simulink model "ModellierungMotor"  (R2014a)
settings: Solver=ode45  StartTime=0.0  StopTime=50  RelTol=1e-3
values from neighbouring files (symbols this model uses):
  Idea = [100000;100]    [DelayDensity_GeneticAlgorithm.m]
  System_A = [0 1 0;0 0 1;0 -C/A -B/A]    [DelayDensity_GeneticAlgorithm.m]
  System_B = [0;0;1/A]    [DelayDensity_GeneticAlgorithm.m]
  System_C = [1 0 0]    [DelayDensity_GeneticAlgorithm.m]
  System_S1 = [0;0;S1/A]    [DelayDensity_GeneticAlgorithm.m]
  System_S2 = [0;0;S2/A]    [DelayDensity_GeneticAlgorithm.m]
  V = -1/(System_C*inv(System_A-System_B*K)*System_B)    [DelayDensity_GeneticAlgorithm.m]
undefined symbols (not defined in the file or in its folder): K, PD, PI, PK
settings Model: Creator=shenc  LastModifiedBy=shenc

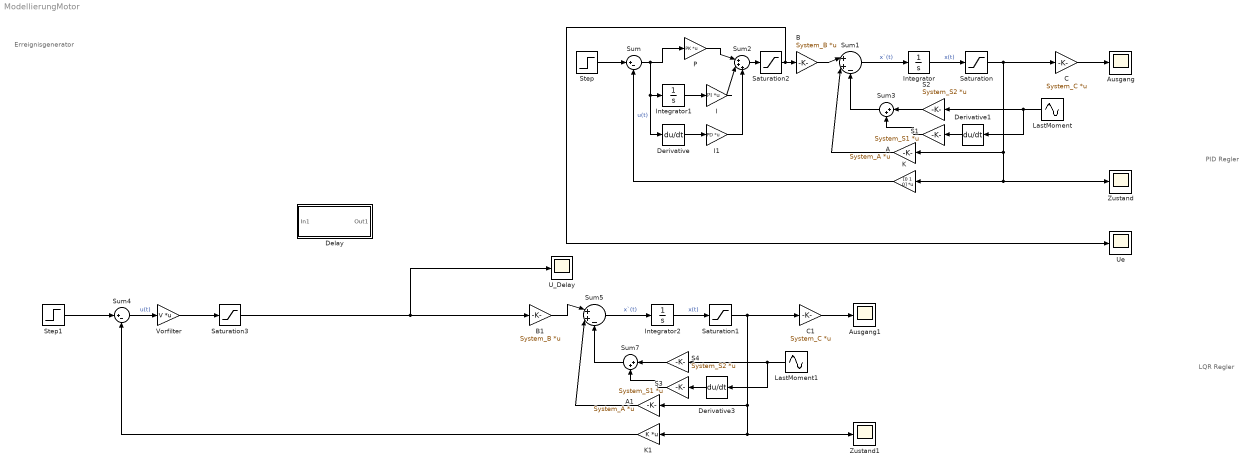
== system ModellierungMotor ==
  note: Erreignisgenerator
  note: LQR Regler
  note: PID Regler
  A : Gain  Gain=System_A  Multiplication=Matrix(K*u)
  A1 : Gain  Gain=System_A  Multiplication=Matrix(K*u)
  Ausgang : Scope
      settings: TimeRange=50  YMin=-2.42338e-27  YMax=5.5e-11
  Ausgang1 : Scope
      settings: TimeRange=50  YMin=-50  YMax=200  SaveName=ScopeData3
  B : Gain  Gain=System_B  Multiplication=Matrix(K*u)
  B1 : Gain  Gain=System_B  Multiplication=Matrix(K*u)
  C : Gain  Gain=System_C  Multiplication=Matrix(K*u)
  C1 : Gain  Gain=System_C  Multiplication=Matrix(K*u)
  Delay : Subsystem
  Derivative : Derivative
  Derivative1 : Derivative
  Derivative3 : Derivative
  I : Gain  Gain=PI  Multiplication=Matrix(K*u)
  I1 : Gain  Gain=PD  Multiplication=Matrix(K*u)
  Integrator : Integrator
  Integrator1 : Integrator
  Integrator2 : Integrator
  K : Gain  Gain=[0 1 0]  Multiplication=Matrix(K*u)
  K1 : Gain  Gain=K  Multiplication=Matrix(K*u)
  LastMoment : Sin  Amplitude=2  SampleTime=0
  LastMoment1 : Sin  Amplitude=2  SampleTime=0
  P : Gain  Gain=PK  Multiplication=Matrix(K*u)
  S1 : Gain  Gain=System_S1  Multiplication=Matrix(K*u)
  S2 : Gain  Gain=System_S2  Multiplication=Matrix(K*u)
  S3 : Gain  Gain=System_S1  Multiplication=Matrix(K*u)
  S4 : Gain  Gain=System_S2  Multiplication=Matrix(K*u)
  Saturation : Saturate  UpperLimit=[500000000 300 500]  LowerLimit=[-500000000 -300 -500]
  Saturation1 : Saturate  UpperLimit=[500000000 300 500]  LowerLimit=[-500000000 -300 -500]
  Saturation2 : Saturate  UpperLimit=1000  LowerLimit=-1000
  Saturation3 : Saturate  UpperLimit=1000  LowerLimit=-1000
  Step : Step  Time=0  After=200  SampleTime=0
  Step1 : Step  Time=0  After=Idea  SampleTime=0
  Sum : Sum  Inputs=|+-
  Sum1 : Sum  Inputs=|++-
  Sum2 : Sum  Inputs=|+++
  Sum3 : Sum  Inputs=|++
  Sum4 : Sum  Inputs=|+-
  Sum5 : Sum  Inputs=|++-
  Sum7 : Sum  Inputs=|++
  U_Delay : Scope
      settings: SaveName=ScopeData6
  Ue : Scope
      settings: TimeRange=50  YMin=-50  YMax=200  SaveName=ScopeData2
  Vorfilter : Gain  Gain=V  Multiplication=Matrix(K*u)
  Zustand : Scope
      settings: YMin=-8.13152e-20  YMax=0.0024
  Zustand1 : Scope
      settings: ShowLegends=on  SaveName=ScopeData5
  wires:
  Sum1/1 -> Integrator/1  "x`(t)"
  B/1 -> Sum1/1
  C/1 -> Ausgang/1
  A/1 -> Sum1/2
  K/1 -> Sum/2
  Step/1 -> Sum/1
  Sum/1 -> Derivative/1, Integrator1/1, P/1  "u(t)"
  P/1 -> Sum2/1
  Integrator1/1 -> I/1
  I/1 -> Sum2/2
  Derivative/1 -> I1/1
  I1/1 -> Sum2/3
  Integrator/1 -> Saturation/1  "x(t)"
  Saturation/1 -> Zustand/1, K/1, A/1, C/1
  LastMoment/1 -> Derivative1/1, S2/1
  Derivative1/1 -> S1/1
  S2/1 -> Sum3/1
  S1/1 -> Sum3/2
  Sum3/1 -> Sum1/3
  Sum5/1 -> Integrator2/1  "x`(t)"
  C1/1 -> Ausgang1/1
  A1/1 -> Sum5/2
  Step1/1 -> Sum4/1
  Integrator2/1 -> Saturation1/1  "x(t)"
  Saturation1/1 -> Zustand1/1, K1/1, A1/1, C1/1
  LastMoment1/1 -> Derivative3/1, S4/1
  Derivative3/1 -> S3/1
  S4/1 -> Sum7/1
  S3/1 -> Sum7/2
  Sum7/1 -> Sum5/3
  Sum4/1 -> Vorfilter/1  "u(t)"
  Sum2/1 -> Saturation2/1
  Saturation2/1 -> Ue/1, B/1
  Vorfilter/1 -> Saturation3/1
  Saturation3/1 -> U_Delay/1, B1/1
  B1/1 -> Sum5/1
  K1/1 -> Sum4/2

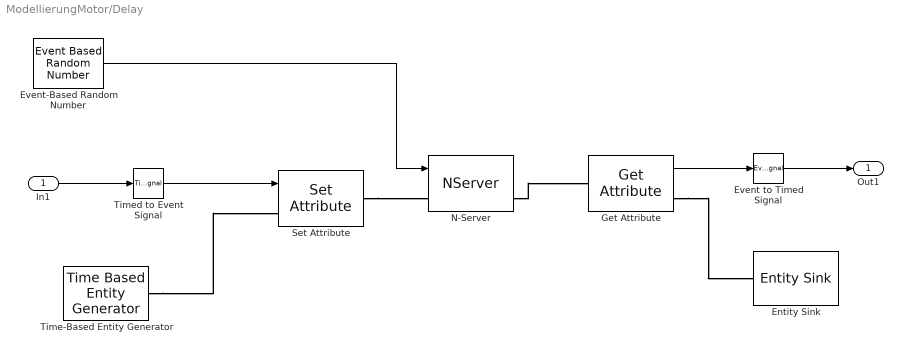
== system ModellierungMotor/Delay ==
  In1 : Inport
  Entity Sink : EntitySink
  Event to Timed Signal : EventToTimedSignal
  Event-Based Random Number : EventBasedRandomNumber  Distribution=Uniform  minUnif=0.1  maxUnif=0.2
  Get Attribute : GetAttribute  AttributeName=Value  EvaluatedDefaultAttributeValue={ []}
      settings: OutputPortMap=o1
  N-Server : NServer  NumberOfServers=1  ServiceTimeFrom=Signal port t  StatNumberDeparted=on
  Set Attribute : SetAttribute  AttributeName=Value  AttributeFrom=Signal port  EvaluatedAttributeValue={ []}
  Time-Based Entity Generator : TimeBasedEntityGenerator  Period=0.01
  Timed to Event Signal : TimedToEventSignal
  Out1 : Outport
  wires:
  In1/1 -> Timed to Event Signal/1
  Event-Based Random Number/1 -> N-Server/1
  Get Attribute/1 -> Event to Timed Signal/1
  Event to Timed Signal/1 -> Out1/1
  Timed to Event Signal/1 -> Set Attribute/1
  connections:
  Time-Based Entity Generator/RConn1 -- Set Attribute/LConn1
  Set Attribute/RConn1 -- N-Server/LConn1
  N-Server/RConn1 -- Get Attribute/LConn1
  Get Attribute/RConn1 -- Entity Sink/LConn1
